simulink model "simulate_FM_Passband_RX"  (R2021a)
settings: Solver=VariableStepAuto  StartTime=0.0  StopTime=0.1  RelTol=1e-3
InitFcn:
  | fs=4e3;
  | Ts=1/fs;
  | frameSize=1;
  | freqDev=250;
libraries: commanapbnd3 x1, dspsrcs4 x1, simulink x1
settings Model: Creator=Byung-Jun Jang  LastModifiedBy=user
settings SolverCC: AlgebraicLoopSolver=TrustRegion
settings DataIOCC: ReturnWorkspaceOutputs=off
settings DebuggingCC: SFMachineParentedDataDiag=warning  ArithmeticOperatorsInVariantConditions=warning
settings SFSimCC: SimUseLocalCustomCode=off  CustomCodeUndefinedFunction=UseInterfaceOnly
settings RTWCC: RTWUseLocalCustomCode=off
settings CodeAppCC: StateflowObjectComments=on
settings SimscapeCC: SimscapeNormalizeSystem=off

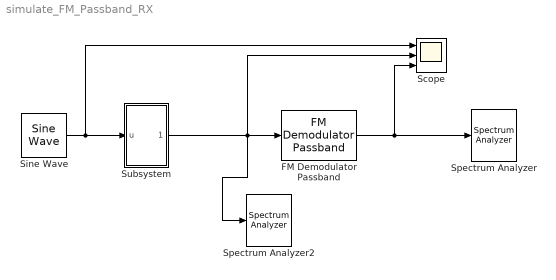
== system simulate_FM_Passband_RX ==
  FM Demodulator Passband : commanapbnd3/FM Demodulator Passband  Fc=1000  Ph=0  Kc=250  Ho=100
      settings: SourceProductBaseCode=CM
  Scope : Scope  NumInputPorts=3
  Sine Wave : dspsrcs4/Sine Wave  Amplitude=1  Frequency=300  Phase=0  SampleMode=Discrete  OutComplex=Real  CompMethod=Trigonometric fcn  TableSize=Speed  SampleTime=1/(fs*10)  SamplesPerFrame=frameSize  ResetState=Restart at time zero  OutputFrames=off  dataType=double  wordLen=16  udDataType=sfix(16)  fracBitsMode=Best precision  numFracBits=15  OutDataTypeStr=double  LastOutDataTypeStr=double
  Spectrum Analyzer : SpectrumAnalyzer
  Spectrum Analyzer2 : SpectrumAnalyzer
  Subsystem : Subsystem
  wires:
  Sine Wave/1 -> Subsystem/1(u), Scope/1
  FM Demodulator Passband/1 -> Scope/3, Spectrum Analyzer/1
  Subsystem/1(Out1) -> Spectrum Analyzer2/1, Scope/2, FM Demodulator Passband/1

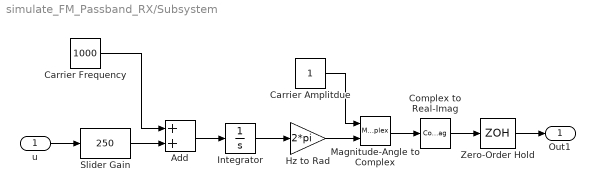
== system simulate_FM_Passband_RX/Subsystem ==
  u : Inport
  Add : Sum
  Carrier Amplitdue : Constant
  Carrier Frequency : Constant  Value=1000
  Complex to Real-Imag : ComplexToRealImag  Output=Real
  Hz to Rad : Gain  Gain=2*pi
  Integrator : Integrator
  Magnitude-Angle to Complex : MagnitudeAngleToComplex
  Slider Gain : simulink/Math Operations/Slider Gain  gain=250  low=0  high=600
      settings: AttributesFormatString=|
      | Frequency
      | Sensitivity
  Zero-Order Hold : ZeroOrderHold  SampleTime=-1
  Out1 : Outport
  wires:
  Magnitude-Angle to Complex/1 -> Complex to Real-Imag/1
  Hz to Rad/1 -> Magnitude-Angle to Complex/2
  Carrier Frequency/1 -> Add/1
  Slider Gain/1 -> Add/2
  Carrier Amplitdue/1 -> Magnitude-Angle to Complex/1
  u/1 -> Slider Gain/1
  Add/1 -> Integrator/1
  Complex to Real-Imag/1 -> Zero-Order Hold/1
  Zero-Order Hold/1 -> Out1/1
  Integrator/1 -> Hz to Rad/1
